simulink model "CaptAxeModeleAvionNonLineaireDiscret"  (R2025b)
settings: Solver=FixedStepDiscrete  StartTime=0.0  StopTime=400  FixedStep=Ts  RelTol=1e-3  EnableMultiTasking=on
values from neighbouring files (symbols this model uses):
  commande_cap = 90    [startCADV.m]
  commande_route = 90    [startCADV.m]
  DEG2RAD = pi/180    (= 0.0174532925199)    [startCADV.m]    (also in stca.m; stcc.m; stcr.m)
  g = 9.80665    [startCADV.m]
  gammae = 0*DEG2RAD    (= 0)    [startCADV.m]
  k = KTS2MS /(2*FL2M)    (= 0.00843904928551)    [startCADV.m]
  k1 = w0^2 * Ve / g    (= 0.0681963542879)    [startCADV.m]
  k11 = 0.1    [startCADV.m]
  k2 = 2*m*w0    (= 0.18)    [startCADV.m]
  k22 = 1    [startCADV.m]
  KTS2MS = NM2M / 3600    (= 0.514444444444)    [startCADV.m]    (also in stca.m = 0.514444)
  phie = 0*5*DEG2RAD    (= 0)    [startCADV.m]
  psie = 0*DEG2RAD    (= 0)    [startCADV.m]
  psiW = 100*DEG2RAD    (= 1.74532925199)    [startCADV.m]
  rhoa = 120*DEG2RAD    (= 2.09439510239)    [startCADV.m]
  tau_ey = 5*tau_psi    (= 50)    [startCADV.m]
  tau_phi = 1    [startCADV.m]
  tau_psi = 10*tau_phi    (= 10)    [startCADV.m]
  tauh = 5*tauGamma    (= 34.098177144)    [startCADV.m]
  Ve = Vie + k*ze    (= 66.8777777778)    [startCADV.m]
  Vie = 130*KTS2MS    (= 66.8777777778)    [startCADV.m]
  W = 30*KTS2MS    (= 15.4333333333)    [startCADV.m]
  xa = 4000    [startCADV.m]
  ya = 3500    [startCADV.m]
  ze = 0*100*FL2M    (= 0)    [startCADV.m]
undefined symbols (not defined in the file or in its folder): DiscIntNeverNeededParam
settings Model: Creator=thierry  LastModifiedBy=vitor
settings SolverCC: AlgebraicLoopSolver=TrustRegion
settings DataIOCC: LimitDataPoints=on  SaveFormat=Array  ReturnWorkspaceOutputs=off
settings OptimizationCC: LifeSpan=inf
settings DebuggingCC: UnderspecifiedInitializationDetection=Classic  MergeDetectMultiDrivingBlocksExec=none  UnconnectedInputMsg=warning  UnconnectedOutputMsg=warning  UnconnectedLineMsg=warning  StateNameClashWarn=warning  SFUnexpectedBacktrackingDiag=warning  SFNoUnconditionalDefaultTransitionDiag=warning  SFExecutionAtInitializationDiag=none  ArithmeticOperatorsInVariantConditions=warning
settings HardwareCC: ProdBitPerPointer=32.0  ProdBitPerSizeT=32.0  ProdBitPerPtrDiffT=32.0  ProdLargestAtomicFloat=None  ProdIntDivRoundTo=Undefined  ProdEndianess=Unspecified  ProdWordSize=32.0  ProdHWDeviceType=32-bit Generic
settings ModelReferenceCC: EnableRefExpFcnMdlSchedulingChecks=on  PropagateSignalLabelsOutOfModel=off
settings SFSimCC: SimUseLocalCustomCode=off  CustomCodeUndefinedFunction=UseInterfaceOnly
settings RTWCC: RTWUseLocalCustomCode=off  GPUComputeCapability=3.5
settings CodeAppCC: StateflowObjectComments=on
settings GRTTargetCC: TargetLangStandard=C89/C90 (ANSI)
settings ConfigComp: CovMetricSettings=dw  CovSaveCumulativeToWorkspaceVar=on  CovSaveSingleToWorkspaceVar=on  CovExternalEMLEnable=off

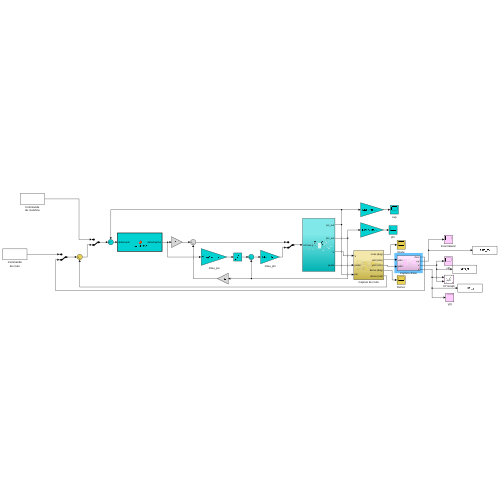
[thumbnail: Simulink's stored preview of the top-level diagram]
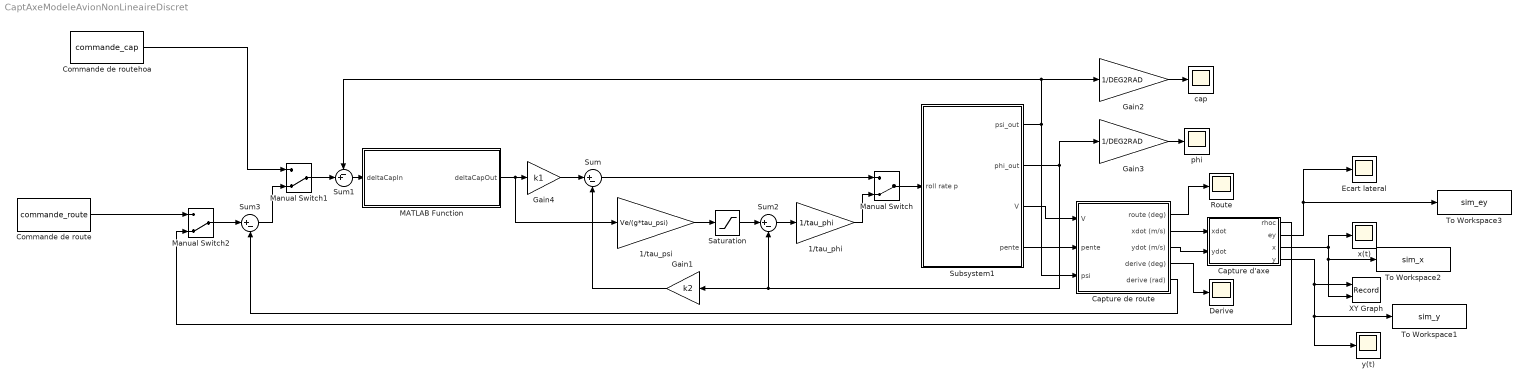
== system CaptAxeModeleAvionNonLineaireDiscret ==
  1/tau_phi : Gain  Gain=1/tau_phi
  1/tau_psi : Gain  Gain=Ve/(g*tau_psi)
  Capture d'axe : Subsystem
  Capture de route : Subsystem
  Commande de route : Constant  Value=commande_route
  Commande de routehoa : Constant  Value=commande_cap
  Derive : Scope
      settings: ActiveDisplayYMinimum=-15.081164763955417  ActiveDisplayYMaximum=11.154001169828421  DataLoggingVariableName=ScopeData3
  Ecart lateral : Scope
      settings: ActiveDisplayYMinimum=-34031.926449064966  ActiveDisplayYMaximum=306287.33804158476  DataLoggingVariableName=ScopeData4
  Gain1 : Gain  Gain=k2
  Gain2 : Gain  Gain=1/DEG2RAD
  Gain3 : Gain  Gain=1/DEG2RAD
  Gain4 : Gain  Gain=k1
  MATLAB Function : MATLAB Function  TreatAsAtomicUnit=on
  Manual Switch : ManualSwitch  CurrentSetting=0
  Manual Switch1 : ManualSwitch  CurrentSetting=0
  Manual Switch2 : ManualSwitch  CurrentSetting=0
  Route : Scope
      settings: ActiveDisplayYMinimum=-133.45616003419806  ActiveDisplayYMaximum=1.2116789248389637  DataLoggingVariableName=ScopeData2
  Saturation : Saturate  UpperLimit=15*DEG2RAD  LowerLimit=-15*DEG2RAD
  Subsystem1 : Subsystem
  Sum : Sum  Inputs=|+-
  Sum1 : Sum  Inputs=-+|
  Sum2 : Sum  Inputs=|+-
  Sum3 : Sum  Inputs=|+-
  To Workspace1 : ToWorkspace  VariableName=sim_y  SaveFormat=Timeseries  SampleTime=-1
  To Workspace2 : ToWorkspace  VariableName=sim_x  SaveFormat=Timeseries  SampleTime=-1
  To Workspace3 : ToWorkspace  VariableName=sim_ey  SaveFormat=Timeseries  SampleTime=-1
  XY Graph : Record  NumPorts=2.0  FileSettingsInternal="{\"entries\":[{\"content\":{\"excelSettings\":{\"content\":{},\"type\":\"Streamout.ExcelSettings\"},\"parquetSettings\":{\"content\":{},\"type\":\"Streamout.ParquetSettings\"}},\"type\":\"Streamout.FileSettingStorage\",\"uuid\":\"\"}],\"packageUris\":[\"http:\\/\\/schema.mathworks.com\\/mf0\\/streamout_blocks\\/R2020a\"],\"version\":\"1.0\"}"  FrameSettings=[0, 0]  Layout=[1 1]  SignalsInternal="{\"entries\":[{\"content\":{\"signals\":[{\"content\":{\"blockPath\":[],\"dimensions\":[1],\"domain\":\"\",\"lineColor\":\"#a2142f\",\"plots\":[ 1 ],\"port\":1,\"sid\":[\"\"],\"signalID\":1,\"signalName\":\"Capture d'axe:4\"},\"type\":\"RecordBlkView.Signal\",\"uuid\":\"\"},{\"content\":{\"blockPath\":[],\"dimensions\":[1],\"domain\":\"\",\"lineColor\":\"#139fff\",\"plots\":[ 1 ],\"port\":2,\"sid\":[\"\"],\"signalID\":2,\"signalName\":\"Capture d'axe:3\"},\"type\":\"RecordBlkView.Signal\",\"uuid\":\"\"}]},\"type\":\"RecordBlkView.InputSignals\",\"uuid\":\"\"}],\"packageUris\":[\"http:\\/\\/schema.mathworks.com\\/mf0\\/streamout_blocks\\/R2020a\"],\"version\":\"1.0\"}"  VisualizationBindings="{\"xyplotplugin\":{\"info\":[{\"series\":[{\"bindingParametersList\":[{\"parameter\":\"X-Axis\",\"signalID\":1,\"signalName\":\"Capture d'axe:4\"},{\"parameter\":\"Y-Axis\",\"signalID\":2,\"signalName\":\"Capture d'axe:3\"}],\"seriesID\":0}],\"subplotID\":1}]}}"  CompatibilityTag=XY
  cap : Scope
      settings: ActiveDisplayYMinimum=-144.80303082336096  ActiveDisplayYMaximum=17.922431645748464  DataLoggingVariableName=ScopeData2
  phi : Scope
      settings: ActiveDisplayYMinimum=-35.842140746185393  ActiveDisplayYMaximum=4.0475505494690314  DataLoggingVariableName=ScopeData3
  x(t) : Scope
      settings: ActiveDisplayYMinimum=-1  ActiveDisplayYMaximum=1  DataLoggingVariableName=ScopeData6
  y(t) : Scope
      settings: ActiveDisplayYMinimum=-1  ActiveDisplayYMaximum=1  DataLoggingVariableName=ScopeData5
  wires:
  Subsystem1/2(phi_out) -> Sum2/2, Gain1/1, Gain3/1
  Gain1/1 -> Sum/2
  Sum1/1 -> MATLAB Function/1(deltaCapIn)
  Subsystem1/1(psi_out) -> Sum1/1, Gain2/1, Capture de route/3(psi)
  Gain2/1 -> cap/1
  Gain3/1 -> phi/1
  Gain4/1 -> Sum/1
  Manual Switch/1 -> Subsystem1/1(roll rate p)
  Sum/1 -> Manual Switch/1
  1/tau_phi/1 -> Manual Switch/2
  Sum2/1 -> 1/tau_phi/1
  Saturation/1 -> Sum2/1
  1/tau_psi/1 -> Saturation/1
  MATLAB Function/1(deltaCapOut) -> 1/tau_psi/1, Gain4/1
  Subsystem1/3(V) -> Capture de route/1(V)
  Subsystem1/4(pente) -> Capture de route/2(pente)
  Capture de route/1(route (deg)) -> Route/1
  Capture de route/4(derive (deg)) -> Derive/1
  Manual Switch1/1 -> Sum1/2
  Commande de routehoa/1 -> Manual Switch1/1
  Sum3/1 -> Manual Switch1/2
  Capture de route/5(derive (rad)) -> Sum3/2
  Commande de route/1 -> Manual Switch2/1
  Capture de route/2(xdot (m/s)) -> Capture d'axe/1(xdot)
  Capture de route/3(ydot (m/s)) -> Capture d'axe/2(ydot)
  Capture d'axe/1(rhoc) -> Manual Switch2/2
  Manual Switch2/1 -> Sum3/1
  Capture d'axe/2(ey) -> To Workspace3/1, Ecart lateral/1
  Capture d'axe/3(x) -> To Workspace2/1, XY Graph/2, x(t)/1
  Capture d'axe/4(y) -> To Workspace1/1, y(t)/1, XY Graph/1

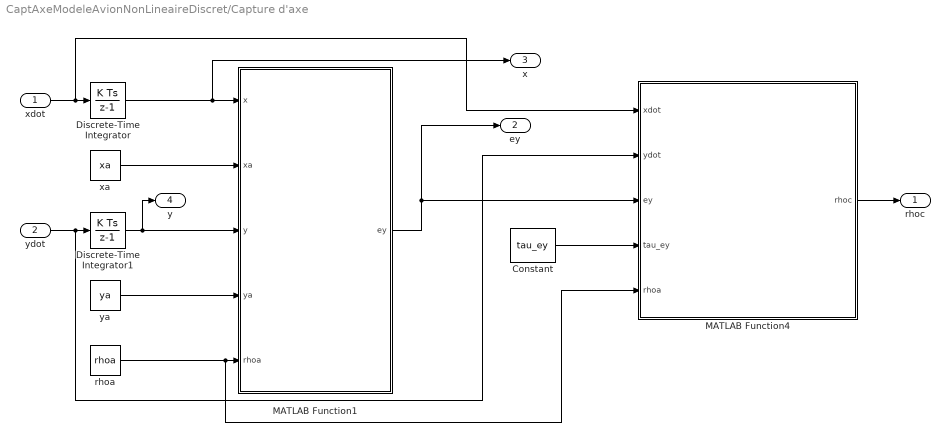
== system CaptAxeModeleAvionNonLineaireDiscret/Capture d'axe ==
  xdot : Inport
  ydot : Inport  Port=2
  Constant : Constant  Value=tau_ey
  Discrete-Time Integrator : DiscreteIntegrator  SampleTime=-1  ICPrevOutput=DiscIntNeverNeededParam  ICPrevScaledInput=DiscIntNeverNeededParam
  Discrete-Time Integrator1 : DiscreteIntegrator  SampleTime=-1  ICPrevOutput=DiscIntNeverNeededParam  ICPrevScaledInput=DiscIntNeverNeededParam
  MATLAB Function1 : MATLAB Function  TreatAsAtomicUnit=on
  MATLAB Function4 : MATLAB Function  TreatAsAtomicUnit=on
  rhoa : Constant  Value=rhoa
  xa : Constant  Value=xa
  ya : Constant  Value=ya
  rhoc : Outport
  ey : Outport  Port=2
  x : Outport  Port=3
  y : Outport  Port=4
  wires:
  MATLAB Function1/1(ey) -> ey/1, MATLAB Function4/3(ey)
  Discrete-Time Integrator1/1 -> y/1, MATLAB Function1/3(y)
  Discrete-Time Integrator/1 -> MATLAB Function1/1(x), x/1
  ydot/1 -> MATLAB Function4/2(ydot), Discrete-Time Integrator1/1
  ya/1 -> MATLAB Function1/4(ya)
  xdot/1 -> Discrete-Time Integrator/1, MATLAB Function4/1(xdot)
  xa/1 -> MATLAB Function1/2(xa)
  Constant/1 -> MATLAB Function4/4(tau_ey)
  rhoa/1 -> MATLAB Function4/5(rhoa), MATLAB Function1/5(rhoa)
  MATLAB Function4/1(rhoc) -> rhoc/1

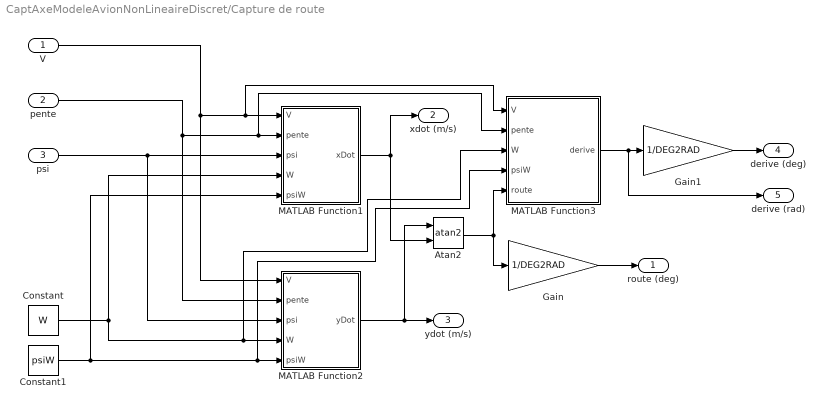
== system CaptAxeModeleAvionNonLineaireDiscret/Capture de route ==
  V : Inport
  pente : Inport  Port=2
  psi : Inport  Port=3
  Atan2 : Trigonometry  Operator=atan2
  Constant : Constant  Value=W
  Constant1 : Constant  Value=psiW
  Gain : Gain  Gain=1/DEG2RAD
  Gain1 : Gain  Gain=1/DEG2RAD
  MATLAB Function1 : MATLAB Function  TreatAsAtomicUnit=on
  MATLAB Function2 : MATLAB Function  TreatAsAtomicUnit=on
  MATLAB Function3 : MATLAB Function  TreatAsAtomicUnit=on
  route (deg) : Outport  VectorParamsAs1DForOutWhenUnconnected=off
  xdot (m/s) : Outport  Port=2  VectorParamsAs1DForOutWhenUnconnected=off
  ydot (m/s) : Outport  Port=3  VectorParamsAs1DForOutWhenUnconnected=off
  derive (deg) : Outport  Port=4  VectorParamsAs1DForOutWhenUnconnected=off
  derive (rad) : Outport  Port=5  VectorParamsAs1DForOutWhenUnconnected=off
  wires:
  pente/1 -> MATLAB Function2/2(pente), MATLAB Function1/2(pente), MATLAB Function3/2(pente)
  V/1 -> MATLAB Function1/1(V), MATLAB Function3/1(V), MATLAB Function2/1(V)
  Constant1/1 -> MATLAB Function2/5(psiW), MATLAB Function3/4(psiW), MATLAB Function1/5(psiW)
  psi/1 -> MATLAB Function2/3(psi), MATLAB Function1/3(psi)
  Atan2/1 -> MATLAB Function3/5(route), Gain/1
  Constant/1 -> MATLAB Function2/4(W), MATLAB Function3/3(W), MATLAB Function1/4(W)
  Gain/1 -> route (deg)/1
  MATLAB Function3/1(derive) -> derive (rad)/1, Gain1/1
  Gain1/1 -> derive (deg)/1
  MATLAB Function2/1(yDot) -> ydot (m/s)/1, Atan2/1
  MATLAB Function1/1(xDot) -> xdot (m/s)/1, Atan2/2

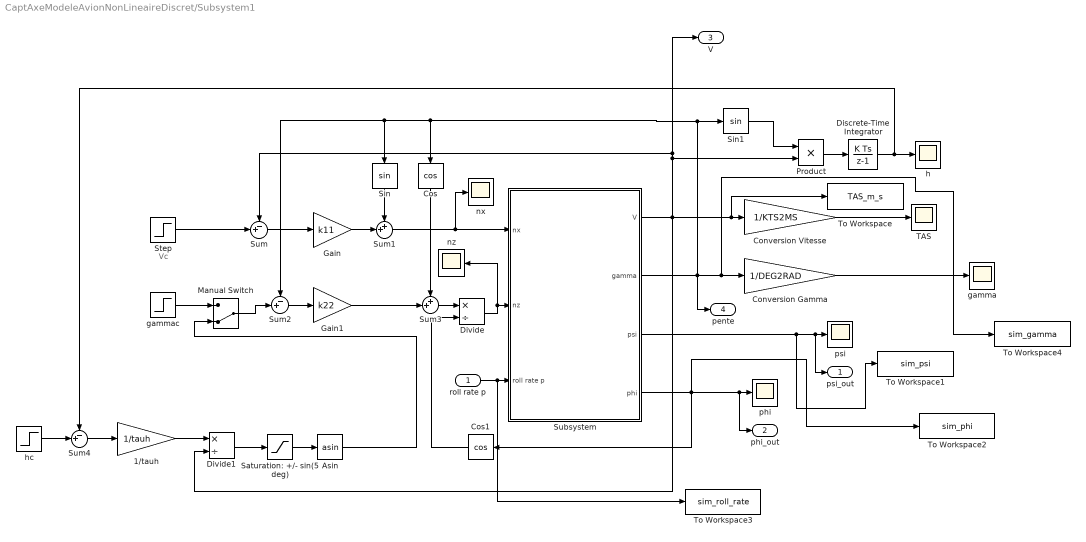
== system CaptAxeModeleAvionNonLineaireDiscret/Subsystem1 ==
  note: Vc
  roll rate p : Inport
  1/tauh : Gain  Gain=1/tauh
  Asin : Trigonometry  Operator=asin
  Conversion Gamma : Gain  Gain=1/DEG2RAD
  Conversion Vitesse : Gain  Gain=1/KTS2MS
  Cos : Trigonometry  Operator=cos
  Cos1 : Trigonometry  Operator=cos
  Discrete-Time Integrator : DiscreteIntegrator  SampleTime=-1  ICPrevOutput=DiscIntNeverNeededParam  ICPrevScaledInput=DiscIntNeverNeededParam
  Divide : Product  Inputs=*/
  Divide1 : Product  Inputs=*/
  Gain : Gain  Gain=k11
  Gain1 : Gain  Gain=k22
  Manual Switch : ManualSwitch  CurrentSetting=0
  Product : Product
  Saturation: +/- sin(5 deg) : Saturate  UpperLimit=sin(5*DEG2RAD)  LowerLimit=-sin(5*DEG2RAD)
  Sin : Trigonometry
  Sin1 : Trigonometry
  Step : Step  Time=0  Before=Ve  After=Ve  SampleTime=0
  Subsystem : Subsystem
  Sum : Sum  Inputs=-+|
  Sum1 : Sum  Inputs=++|
  Sum2 : Sum  Inputs=-+|
  Sum3 : Sum  Inputs=++|
  Sum4 : Sum  Inputs=-+|
  TAS : Scope
      settings: ActiveDisplayYMinimum=-1  ActiveDisplayYMaximum=1
  To Workspace : ToWorkspace  VariableName=TAS_m_s  SaveFormat=Timeseries  SampleTime=-1
  To Workspace1 : ToWorkspace  VariableName=sim_psi  SaveFormat=Timeseries  SampleTime=-1
  To Workspace2 : ToWorkspace  VariableName=sim_phi  SaveFormat=Timeseries  SampleTime=-1
  To Workspace3 : ToWorkspace  VariableName=sim_roll_rate  SaveFormat=Timeseries  SampleTime=-1
  To Workspace4 : ToWorkspace  VariableName=sim_gamma  SaveFormat=Timeseries  SampleTime=-1
  gamma : Scope
      settings: ActiveDisplayYMinimum=-1  ActiveDisplayYMaximum=1
  "gammac " : Step  Time=10  After=3*DEG2RAD  SampleTime=0
  h : Scope
      settings: ActiveDisplayYMinimum=-2.8E-13  ActiveDisplayYMaximum=3E-14
  hc : Step  Time=0  After=0  SampleTime=0
  nx : Scope
      settings: ActiveDisplayYMinimum=-1.1E-16  ActiveDisplayYMaximum=1.2E-16
  nz : Scope
      settings: ActiveDisplayYMinimum=0.99758  ActiveDisplayYMaximum=1.03661
  phi : Scope
      settings: ActiveDisplayYMinimum=-1  ActiveDisplayYMaximum=1  DataLoggingVariableName=ScopeData3
  psi : Scope
      settings: ActiveDisplayYMinimum=-0.39361  ActiveDisplayYMaximum=3.54245  DataLoggingVariableName=ScopeData2
  psi_out : Outport  VectorParamsAs1DForOutWhenUnconnected=off
  phi_out : Outport  Port=2  VectorParamsAs1DForOutWhenUnconnected=off
  V : Outport  Port=3  VectorParamsAs1DForOutWhenUnconnected=off
  pente : Outport  Port=4  VectorParamsAs1DForOutWhenUnconnected=off
  wires:
  Sum2/1 -> Gain1/1
  Step/1 -> Sum/2
  Discrete-Time Integrator/1 -> Sum4/1, h/1
  Subsystem/2(gamma) -> pente/1, To Workspace4/1, Conversion Gamma/1, Sum2/1, Sin/1, Cos/1, Sin1/1
  Sum/1 -> Gain/1
  1/tauh/1 -> Divide1/1
  Subsystem/3(psi) -> To Workspace1/1, psi_out/1, psi/1
  Divide1/1 -> Saturation: +/- sin(5 deg)/1
  Subsystem/1(V) -> Divide1/2, To Workspace/1, Conversion Vitesse/1, V/1, Sum/1, Product/2
  hc/1 -> Sum4/2
  Divide/1 -> nz/1, Subsystem/2(nz)
  Subsystem/4(phi) -> To Workspace2/1, phi_out/1, phi/1, Cos1/1
  Asin/1 -> Manual Switch/2
  roll rate p/1 -> To Workspace3/1, Subsystem/3(roll rate p)
  Cos1/1 -> Divide/2
  Sin/1 -> Sum1/1
  Conversion Gamma/1 -> gamma/1
  Cos/1 -> Sum3/1
  Sum1/1 -> nx/1, Subsystem/1(nx)
  Gain/1 -> Sum1/2
  Sum4/1 -> 1/tauh/1
  "gammac "/1 -> Manual Switch/1
  Product/1 -> Discrete-Time Integrator/1
  Sum3/1 -> Divide/1
  Saturation: +/- sin(5 deg)/1 -> Asin/1
  Manual Switch/1 -> Sum2/2
  Gain1/1 -> Sum3/2
  Sin1/1 -> Product/1
  Conversion Vitesse/1 -> TAS/1

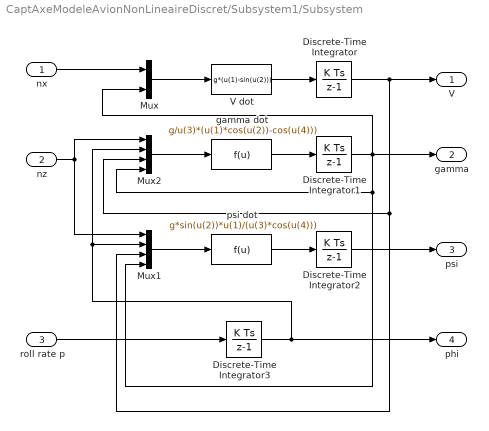
== system CaptAxeModeleAvionNonLineaireDiscret/Subsystem1/Subsystem ==
  nx : Inport
  nz : Inport  Port=2
  roll rate p : Inport  Port=3
  Discrete-Time Integrator : DiscreteIntegrator  InitialCondition=Vie + k*ze  SampleTime=-1  ICPrevOutput=DiscIntNeverNeededParam  ICPrevScaledInput=DiscIntNeverNeededParam
  Discrete-Time Integrator1 : DiscreteIntegrator  InitialCondition=gammae  SampleTime=-1  ICPrevOutput=DiscIntNeverNeededParam  ICPrevScaledInput=DiscIntNeverNeededParam
  Discrete-Time Integrator2 : DiscreteIntegrator  InitialCondition=psie  SampleTime=-1  ICPrevOutput=DiscIntNeverNeededParam  ICPrevScaledInput=DiscIntNeverNeededParam
  Discrete-Time Integrator3 : DiscreteIntegrator  InitialCondition=phie  SampleTime=-1  ICPrevOutput=DiscIntNeverNeededParam  ICPrevScaledInput=DiscIntNeverNeededParam
  Mux : Mux  Inputs=2
  Mux1 : Mux
  Mux2 : Mux
  V dot : Fcn  Expr=g*(u(1)-sin(u(2)))
  gamma dot : Fcn  Expr=g/u(3)*(u(1)*cos(u(2))-cos(u(4)))
  psi dot : Fcn  Expr=g*sin(u(2))*u(1)/(u(3)*cos(u(4)))
  V : Outport  VectorParamsAs1DForOutWhenUnconnected=off
  gamma : Outport  Port=2  VectorParamsAs1DForOutWhenUnconnected=off
  psi : Outport  Port=3  VectorParamsAs1DForOutWhenUnconnected=off
  phi : Outport  Port=4  VectorParamsAs1DForOutWhenUnconnected=off
  wires:
  roll rate p/1 -> Discrete-Time Integrator3/1
  nx/1 -> Mux/1
  nz/1 -> Mux1/1, Mux2/1
  Mux2/1 -> gamma dot/1
  Discrete-Time Integrator3/1 -> phi/1, Mux1/2, Mux2/2
  Mux/1 -> V dot/1
  psi dot/1 -> Discrete-Time Integrator2/1
  Discrete-Time Integrator2/1 -> psi/1
  Mux1/1 -> psi dot/1
  gamma dot/1 -> Discrete-Time Integrator1/1
  Discrete-Time Integrator/1 -> V/1, Mux2/3, Mux1/3
  V dot/1 -> Discrete-Time Integrator/1
  Discrete-Time Integrator1/1 -> gamma/1, Mux/2, Mux2/4, Mux1/4

== matlab function CaptAxeModeleAvionNonLineaireDiscret/Capture de route/MATLAB Function1 ==
  data: V input; xDot output; pente input; psi input; W input; psiW input
function xDot = xDotFcn(V, pente, psi, W, psiW)

xDot = V*cos(pente)*cos(psi) + W*cos(psiW + pi);

== matlab function CaptAxeModeleAvionNonLineaireDiscret/MATLAB Function ==
  data: deltaCapIn input; deltaCapOut output
function deltaCapOut = modulo360(deltaCapIn)

deltaCapOut = deltaCapIn;
while (deltaCapOut > pi)
    deltaCapOut = deltaCapOut - 2*pi;
end
while (deltaCapOut < -pi)
    deltaCapOut = deltaCapOut + 2*pi;
end

== matlab function CaptAxeModeleAvionNonLineaireDiscret/Capture de route/MATLAB Function2 ==
  data: V input; yDot output; pente input; psi input; W input; psiW input
function yDot = yDotFcn(V, pente, psi, W, psiW)

yDot = V*cos(pente)*sin(psi) + W*sin(psiW + pi);

== matlab function CaptAxeModeleAvionNonLineaireDiscret/Capture d'axe/MATLAB Function1 ==
  data: x input; ey output; xa input; y input; ya input; rhoa input
function ey = captureEcartLateral(x, xa, y, ya, rhoa)

ey = -(x - xa) * sin(rhoa) + (y - ya) * cos(rhoa);

== matlab function CaptAxeModeleAvionNonLineaireDiscret/Capture de route/MATLAB Function3 ==
  data: V input; derive output; pente input; W input; psiW input; route input
function derive = deriveFcn(V, pente, W, psiW, route)

argSin = W/(V*cos(pente))*sin(pi + psiW - route);
if argSin > 1
    argSin = 1;
elseif argSin < -1
    argSin = -1;
end
derive = asin(argSin);

== matlab function CaptAxeModeleAvionNonLineaireDiscret/Capture d'axe/MATLAB Function4 ==
  data: xdot input; ydot input; ey input; tau_ey input; rhoc output; rhoa input
function rhoc = captureConsigneRhoC_SansEx(xdot, ydot, ey, tau_ey, rhoa)

Gs = sqrt(xdot^2 + ydot^2);

argSin = -ey / (tau_ey * Gs);
if argSin > 1
    argSin = 1;
elseif argSin < -1
    argSin = -1;
end

rhoc = asin(argSin) + rhoa;
